simulink model "pendulum"  (Simulink 7.4)
settings: Solver=ode45  StartTime=0.0  StopTime=5  MaxStep=0.05  RelTol=1e-6
values from neighbouring files (symbols this model uses):
  g = 9.81    [ARI_pendulum.m]
  l = 0.7    [ARI_pendulum.m]
  m = 0.3    [ARI_pendulum.m]
  Mc = 0    [ARI_pendulum.m]
  SP = [0 0 0]    [ARI_pendulum.m]
  x0 = [pi/4 0]    [ARI_pendulum.m]
settings Model: Creator=Chandler  LastModifiedBy=Vana_E11
settings DebuggingCC: StrictBusMsg=ErrorLevel1

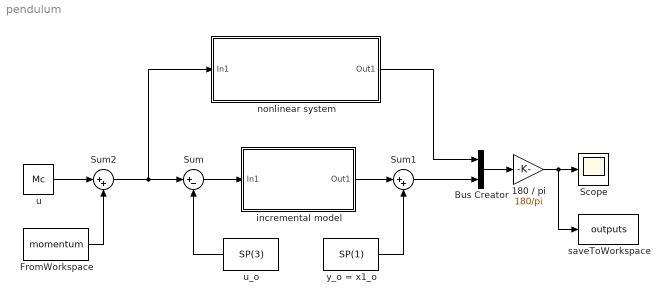
== system pendulum ==
  180 / pi : Gain  Gain=180/pi  ParameterDataType=fixdt(1, 16)  ParameterScaling=2^0  OutDataType=fixdt(1, 16)  OutScaling=2^0
  Bus Creator : BusCreator  Inputs=2
  FromWorkspace : FromWorkspace  VariableName=momentum  SampleTime=0
  Scope : Scope
      settings: TimeRange=5
  Sum : Sum  Inputs=|+-  OutDataType=fixdt(1, 16)  OutScaling=2^0
  Sum1 : Sum  Inputs=|++  OutDataType=fixdt(1, 16)  OutScaling=2^0
  Sum2 : Sum  Inputs=|++  OutDataType=fixdt(1, 16)  OutScaling=2^0
  incremental model : Subsystem
  nonlinear system : Subsystem
  saveToWorkspace : ToWorkspace  VariableName=outputs  SampleTime=-1  SaveFormat=Structure With Time
  u : Constant  Value=Mc  OutDataType=fixdt(1, 16)  OutScaling=2^0
  u_o : Constant  Value=SP(3)  OutDataType=fixdt(1, 16)  OutScaling=2^0
  y_o = x1_o : Constant  Value=SP(1)  OutDataType=fixdt(1, 16)  OutScaling=2^0
  wires:
  Bus Creator/1 -> 180 / pi/1
  180 / pi/1 -> saveToWorkspace/1, Scope/1
  Sum/1 -> incremental model/1(In1)
  y_o = x1_o/1 -> Sum1/2
  u_o/1 -> Sum/2
  incremental model/1(Out1) -> Sum1/1
  Sum1/1 -> Bus Creator/2
  nonlinear system/1(Out1) -> Bus Creator/1
  u/1 -> Sum2/1
  FromWorkspace/1 -> Sum2/2
  Sum2/1 -> Sum/1, nonlinear system/1(In1)

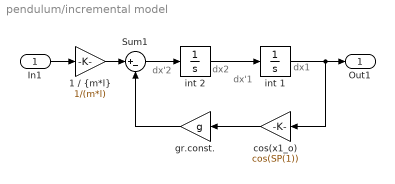
== system pendulum/incremental model ==
  note: dx1
  note: dx'1
  note: dx2
  note: dx'2
  In1 : Inport
  "1 / {m*l}" : Gain  Gain=1/(m*l)  ParameterDataType=fixdt(1, 16)  ParameterScaling=2^0  OutDataType=fixdt(1, 16)  OutScaling=2^0
  Sum1 : Sum  Inputs=|+-  OutDataType=fixdt(1, 16)  OutScaling=2^0
  cos(x1_o) : Gain  Gain=cos(SP(1))  ParameterDataType=fixdt(1, 16)  ParameterScaling=2^0  OutDataType=fixdt(1, 16)  OutScaling=2^0
  gr.const. : Gain  Gain=g  ParameterDataType=fixdt(1, 16)  ParameterScaling=2^0  OutDataType=fixdt(1, 16)  OutScaling=2^0
  int 1 : Integrator  InitialCondition=x0(1)-SP(1)
  int 2 : Integrator  InitialCondition=x0(2)-SP(2)
  Out1 : Outport
  wires:
  int 2/1 -> int 1/1
  int 1/1 -> cos(x1_o)/1, Out1/1
  Sum1/1 -> int 2/1
  gr.const./1 -> Sum1/2
  "1 / {m*l}"/1 -> Sum1/1
  cos(x1_o)/1 -> gr.const./1
  In1/1 -> "1 / {m*l}"/1

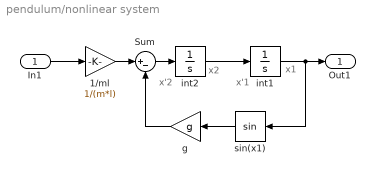
== system pendulum/nonlinear system ==
  note: x1
  note: x2
  note: x'1
  note: x'2
  In1 : Inport
  1/ml : Gain  Gain=1/(m*l)  ParameterDataType=fixdt(1, 16)  ParameterScaling=2^0  OutDataType=fixdt(1, 16)  OutScaling=2^0
  Sum : Sum  Inputs=|+-  OutDataType=fixdt(1, 16)  OutScaling=2^0
  g : Gain  Gain=g  ParameterDataType=fixdt(1, 16)  ParameterScaling=2^0  OutDataType=fixdt(1, 16)  OutScaling=2^0
  int1 : Integrator  InitialCondition=x0(1)
  int2 : Integrator  InitialCondition=x0(2)
  sin(x1) : Trigonometry
  Out1 : Outport
  wires:
  int2/1 -> int1/1
  sin(x1)/1 -> g/1
  int1/1 -> sin(x1)/1, Out1/1
  Sum/1 -> int2/1
  g/1 -> Sum/2
  1/ml/1 -> Sum/1
  In1/1 -> 1/ml/1
